simulink model "simulinkeasy"  (R2016a)
settings: Solver=FixedStepAuto  StartTime=0.0  StopTime=10.0  RelTol=1e-3
settings Model: Creator=Dom  LastModifiedBy=Dominik

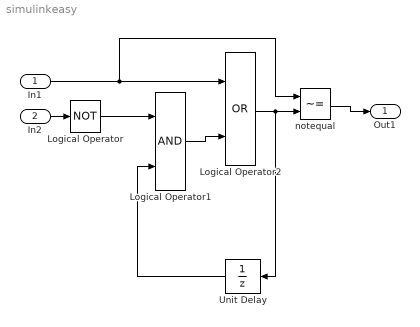
== system simulinkeasy ==
  In1 : Inport
  In2 : Inport  Port=2
  Logical Operator : Logic  Operator=NOT  AllPortsSameDT=off  OutDataTypeStr=boolean
  Logical Operator1 : Logic  AllPortsSameDT=off  OutDataTypeStr=boolean
  Logical Operator2 : Logic  Operator=OR  AllPortsSameDT=off  OutDataTypeStr=boolean
  Unit Delay : UnitDelay  SampleTime=-1
  notequal : RelationalOperator  Operator=~=  OutDataTypeStr=boolean
  Out1 : Outport
  wires:
  In2/1 -> Logical Operator/1
  Logical Operator1/1 -> Logical Operator2/2
  In1/1 -> notequal/1, Logical Operator2/1
  Logical Operator2/1 -> Unit Delay/1, notequal/2
  Unit Delay/1 -> Logical Operator1/2
  Logical Operator/1 -> Logical Operator1/1
  notequal/1 -> Out1/1
